simulink model "discretePIDModel"  (R2025a)
settings: Solver=VariableStepAuto  StartTime=0.0  StopTime=10.0  RelTol=1e-3
model workspace (MAT data in the model file):
  Ts = 0.1
  ki = 1
  kp = 0.2
settings Model: Creator=JPIRES3  LastModifiedBy=JPIRES3

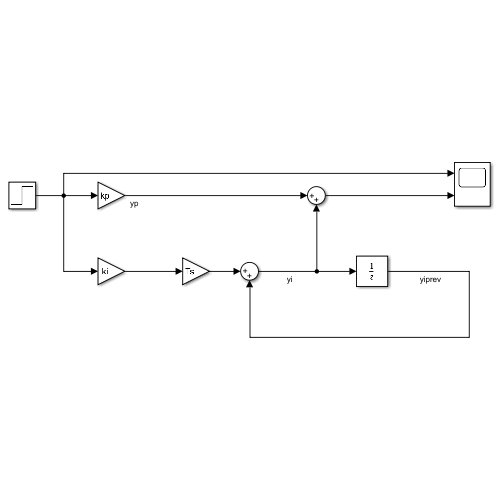
[thumbnail: Simulink's stored preview of the top-level diagram]
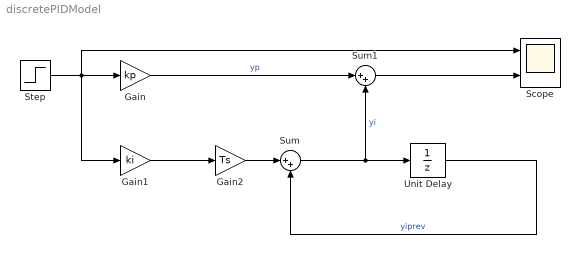
== system discretePIDModel ==
  Gain : Gain  Gain=kp
  Gain1 : Gain  Gain=ki
  Gain2 : Gain  Gain=Ts
  Scope : Scope  NumInputPorts=2
      settings: ActiveDisplayYMinimum=-0.33750000000000013  ActiveDisplayYMaximum=3.0375000000000019
  Step : Step  SampleTime=0
  Sum : Sum  Inputs=|++
  Sum1 : Sum  Inputs=|++
  Unit Delay : UnitDelay  InitialCondition=1  SampleTime=.6  HasFrameUpgradeWarning=on
  wires:
  Step/1 -> Gain1/1, Scope/1, Gain/1
  Gain/1 -> Sum1/1  "yp"
  Unit Delay/1 -> Sum/2  "yiprev"
  Gain1/1 -> Gain2/1
  Gain2/1 -> Sum/1
  Sum/1 -> Sum1/2, Unit Delay/1  "yi"
  Sum1/1 -> Scope/2
